simulink model "t2_sim"  (Simulink 7.3)
settings: Solver=ode45  StartTime=0.0  StopTime=4  RelTol=1e-3
values from neighbouring files (symbols this model uses):
  B = 5    [t1.m]
  K = 50    [t1.m]
  M = 1    [t1.m]
  Ts = .02    (= 0.02)    [t1.m]
settings Model: Creator=arash  LastModifiedBy=arash

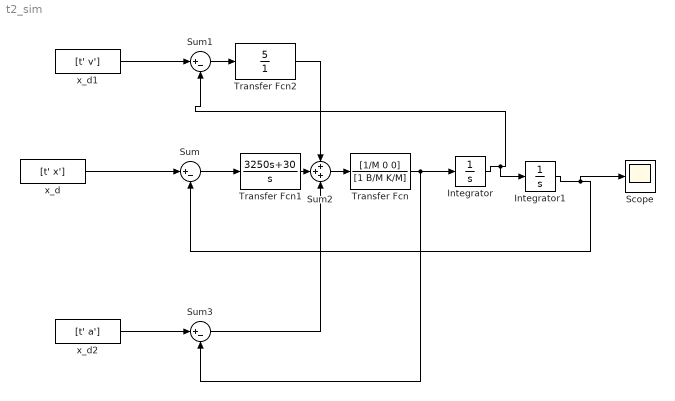
== system t2_sim ==
  Integrator : Integrator
  Integrator1 : Integrator
  Scope : Scope
      settings: TimeRange=15
  Sum : Sum  Inputs=|+-  OutDataType=fixdt(1, 16)  OutScaling=2^0
  Sum1 : Sum  Inputs=|+-  OutDataType=fixdt(1, 16)  OutScaling=2^0
  Sum2 : Sum  Inputs=+++  OutDataType=fixdt(1, 16)  OutScaling=2^0
  Sum3 : Sum  Inputs=|+-  OutDataType=fixdt(1, 16)  OutScaling=2^0
  Transfer Fcn : TransferFcn  Numerator=[1/M 0 0]  Denominator=[1 B/M K/M]
  Transfer Fcn1 : TransferFcn  Numerator=[3250 30]  Denominator=[1 0]
  Transfer Fcn2 : TransferFcn  Numerator=5  Denominator=1
  x_d : FromWorkspace  VariableName=[t' x']  SampleTime=Ts
  x_d1 : FromWorkspace  VariableName=[t' v']  SampleTime=Ts
  x_d2 : FromWorkspace  VariableName=[t' a']  SampleTime=Ts
  wires:
  Sum/1 -> Transfer Fcn1/1
  x_d/1 -> Sum/1
  Transfer Fcn/1 -> Integrator/1, Sum3/2
  Sum2/1 -> Transfer Fcn/1
  Transfer Fcn1/1 -> Sum2/2
  x_d1/1 -> Sum1/1
  Integrator1/1 -> Scope/1, Sum/2
  Integrator/1 -> Sum1/2, Integrator1/1
  x_d2/1 -> Sum3/1
  Sum1/1 -> Transfer Fcn2/1
  Transfer Fcn2/1 -> Sum2/1
  Sum3/1 -> Sum2/3
